simulink model "EMF"  (Simulink 7.4)
settings: Solver=ode45  StartTime=0.0  StopTime=10.0  RelTol=1e-3
settings Model: Creator=dread  LastModifiedBy=dread

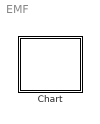
== system EMF ==
  Chart : Stateflow chart

== stateflow chart Chart ==
  state State
    entry: doState()
  (default) -> State
  State -> State : /doTransition()
  function doTransition:
    | function doTransition
    | %doTransition
  function doState:
    | function doState
    | %doState
  function nestedEMF:
    | function nestedEMF
    | %nestedEMF
